simulink model "at40jointmodeltest"  (R2016a)
settings: Solver=VariableStepAuto  StartTime=0.0  StopTime=100  RelTol=1e-3
settings Model: Creator=julianleland  LastModifiedBy=julianleland

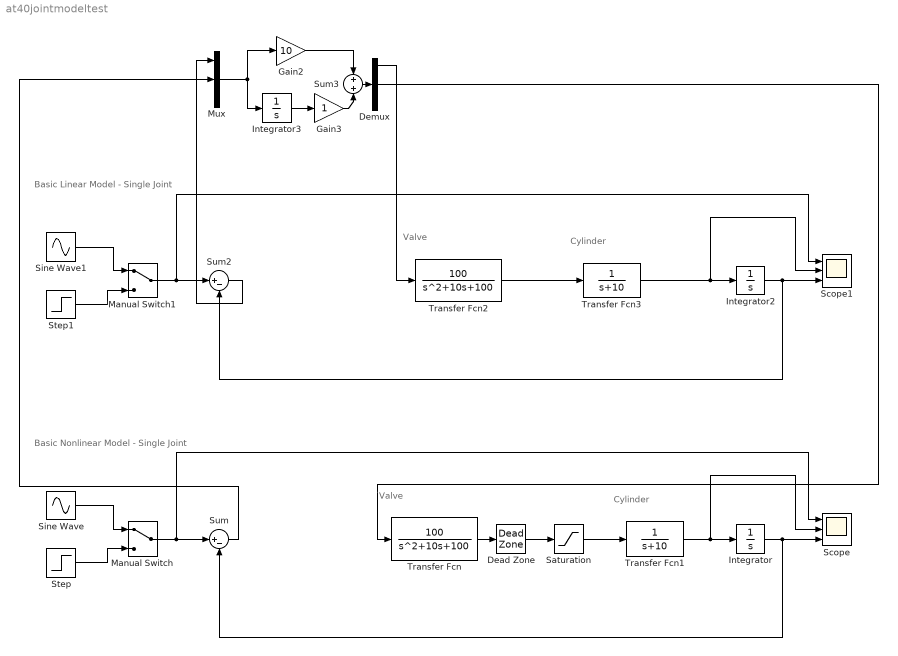
== system at40jointmodeltest ==
  note: Basic Nonlinear Model - Single Joint
  note: Cylinder
  note: Valve
  note: Basic Linear Model - Single Joint
  note: Cylinder
  note: Valve
  Dead Zone : DeadZone  LowerValue=-0.1  UpperValue=0.1  SaturateOnIntegerOverflow=on
  Demux : Demux  Outputs=3
  Gain2 : Gain  Gain=10
  Gain3 : Gain
  Integrator : Integrator  LimitOutput=on  UpperSaturationLimit=10  LowerSaturationLimit=-10
  Integrator2 : Integrator  LimitOutput=on  UpperSaturationLimit=10  LowerSaturationLimit=-10
  Integrator3 : Integrator  LimitOutput=on  UpperSaturationLimit=0.1  LowerSaturationLimit=-0.1
  Manual Switch : ManualSwitch
  Manual Switch1 : ManualSwitch
  Mux : Mux  Inputs=3
  Saturation : Saturate  UpperLimit=0.9  LowerLimit=-0.9
  Scope : Scope  NumInputPorts=3
  Scope1 : Scope  NumInputPorts=3
  Sine Wave : Sin  Amplitude=5  Frequency=0.1  SampleTime=0
  Sine Wave1 : Sin  Amplitude=5  Frequency=0.1  SampleTime=0
  Step : Step  SampleTime=0
  Step1 : Step  SampleTime=0
  Sum : Sum  Inputs=|+-
  Sum2 : Sum  Inputs=|+-
  Sum3 : Sum
  Transfer Fcn : TransferFcn  Numerator=100  Denominator=[1 10 100]
  Transfer Fcn1 : TransferFcn  Denominator=[1 10]
  Transfer Fcn2 : TransferFcn  Numerator=100  Denominator=[1 10 100]
  Transfer Fcn3 : TransferFcn  Denominator=[1 10]
  wires:
  Dead Zone/1 -> Saturation/1
  Saturation/1 -> Transfer Fcn1/1
  Manual Switch/1 -> Scope/1, Sum/1
  Integrator/1 -> Scope/3, Sum/2
  Transfer Fcn/1 -> Dead Zone/1
  Transfer Fcn1/1 -> Scope/2, Integrator/1
  Sine Wave/1 -> Manual Switch/1
  Step/1 -> Manual Switch/2
  Transfer Fcn2/1 -> Transfer Fcn3/1
  Mux/1 -> Integrator3/1, Gain2/1
  Manual Switch1/1 -> Scope1/1, Sum2/1
  Integrator2/1 -> Scope1/3, Sum2/2
  Transfer Fcn3/1 -> Scope1/2, Integrator2/1
  Sine Wave1/1 -> Manual Switch1/1
  Step1/1 -> Manual Switch1/2
  Gain2/1 -> Sum3/1
  Demux/1 -> Transfer Fcn2/1
  Integrator3/1 -> Gain3/1
  Gain3/1 -> Sum3/2
  Sum2/1 -> Mux/1
  Sum/1 -> Mux/2
  Sum3/1 -> Demux/1
  Demux/2 -> Transfer Fcn/1
